simulink model "Test_controlled_3_phase_V_source"  (Simulink 7.7)
settings: Solver=ode45  StartTime=0.0  StopTime=10.0  RelTol=1e-3
libraries: powerlib x7, pm_machines_library x1
settings Model: Creator=s0237326  LastModifiedBy=s0237326

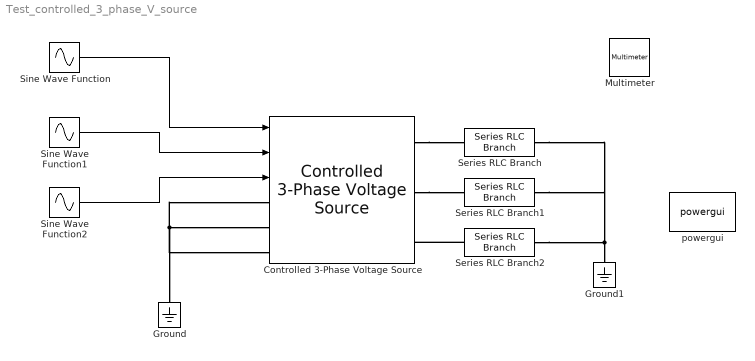
== system Test_controlled_3_phase_V_source ==
  Controlled 3-Phase Voltage Source : pm_machines_library/Controlled 3-Phase Voltage Source  SystemSampleTime=-1
      link override Controlled Voltage Source A: Source_Type=DC  Initialize=off
      link override Controlled Voltage Source C: Source_Type=DC  Initialize=off
      link override Controlled Voltage Source1: Source_Type=DC  Initialize=off
  Ground : powerlib/Elements/Ground  PhysicalDomain=powersysdomain  SubClassName=unknown  LeftPortType=p1  RightPortType=p1  LConnTagsString=a
  Ground1 : powerlib/Elements/Ground  PhysicalDomain=powersysdomain  SubClassName=unknown  LeftPortType=p1  RightPortType=p1  LConnTagsString=a
  Multimeter : powerlib/Measurements/Multimeter  SystemSampleTime=-1  PhasorSimulation=off  OutputType=Complex  sel=[1 4 3 4 5 6]  L=6  Gain=[1 1 1 1 1 1]  yselected={'Ub: Series RLC Branch','Ib: Series RLC Branch','Ub: Series RLC Branch2','Ib: Series RLC Branch','Ib: Series RLC Branch1','Ib: Series RLC Branch2'};  PSBOutputType=1  PSBequivalent=0  AxesSetting=[0,0.1,-100,100]  Display=1  SavedBlockNames=-11
  Series RLC Branch : powerlib/Elements/Series RLC Branch  PhysicalDomain=powersysdomain  SubClassName=unknown  LeftPortType=p1  RightPortType=p1  LConnTagsString=__new0  RConnTagsString=__new0  BranchType=R  Resistance=1  Inductance=0  SetiL0=off  InitialCurrent=0  Capacitance=0  Setx0=off  InitialVoltage=0  Measurements=Branch voltage and current
  Series RLC Branch1 : powerlib/Elements/Series RLC Branch  PhysicalDomain=powersysdomain  SubClassName=unknown  LeftPortType=p1  RightPortType=p1  LConnTagsString=__new0  RConnTagsString=__new0  BranchType=R  Resistance=1  Inductance=1e-3  SetiL0=off  InitialCurrent=0  Capacitance=1e-6  Setx0=off  InitialVoltage=0  Measurements=Branch voltage and current
  Series RLC Branch2 : powerlib/Elements/Series RLC Branch  PhysicalDomain=powersysdomain  SubClassName=unknown  LeftPortType=p1  RightPortType=p1  LConnTagsString=__new0  RConnTagsString=__new0  BranchType=R  Resistance=1  Inductance=1e-3  SetiL0=off  InitialCurrent=0  Capacitance=1e-6  Setx0=off  InitialVoltage=0  Measurements=Branch voltage and current
  Sine Wave Function : Sin  Frequency=6.28  SampleTime=0
  Sine Wave Function1 : Sin  Frequency=6.28  Phase=2.0944  SampleTime=0
  Sine Wave Function2 : Sin  Frequency=6.28  Phase=4.188  SampleTime=0
  powergui : powerlib/powergui  Priority=1  SystemSampleTime=-1  SimulationMode=Continuous  SampleTime=50e-6  frequency=60  SPID=off  DisableSnubberDevices=off  DisableRonSwitches=off  DisableVfSwitches=off  SwTol=0  Interpol=off  DisplayEquations=off  FunctionMessages=off  frequencyindice=0  Pbase=100e6  ErrMax=1e-4  Iterations=50  UnitsV=kV  UnitsW=MW  echomessages=off  HookPort=off  EnableUseOfTLC=off  x0status=blocks  RestoreLinks=warning  ResistiveCurrentMeasurement=off  Ylog=off  Xlog=on  ShowGrid=off  save=off  variable=ZData  ZoomFFT=off  StartTime=0.0  cycles=1  DisplayStyle=1  FreqAxis=off  MaxFrequency=1000  frequencyindicesteady=1  display=off  methode=off
  wires:
  Sine Wave Function/1 -> Controlled 3-Phase Voltage Source/1
  Sine Wave Function1/1 -> Controlled 3-Phase Voltage Source/2
  Sine Wave Function2/1 -> Controlled 3-Phase Voltage Source/3
  connections:
  Ground/LConn1 -- Controlled 3-Phase Voltage Source/LConn3 -- Controlled 3-Phase Voltage Source/LConn1 -- Controlled 3-Phase Voltage Source/LConn2
  Series RLC Branch2/LConn1 -- Controlled 3-Phase Voltage Source/RConn3
  Controlled 3-Phase Voltage Source/RConn2 -- Series RLC Branch1/LConn1
  Controlled 3-Phase Voltage Source/RConn1 -- Series RLC Branch/LConn1
  Series RLC Branch/RConn1 -- Series RLC Branch1/RConn1 -- Ground1/LConn1 -- Series RLC Branch2/RConn1
